simulink model "LinearMPCsiso"  (R2020b)
settings: Solver=FixedStepDiscrete  StartTime=0.0  StopTime=10.0  FixedStep=0.05  RelTol=1e-3
settings Model: Creator=iris  LastModifiedBy=iris
settings DebuggingCC: SFMachineParentedDataDiag=error

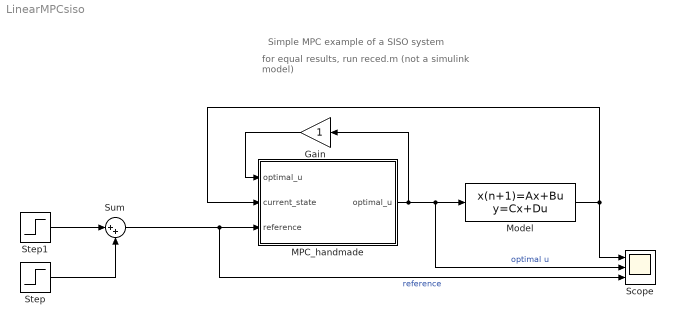
== system LinearMPCsiso ==
  note: for equal results, run reced.m (not a simulink model)
  note: Simple MPC example of a SISO system
  Gain : Gain
  MPC_handmade : MATLAB Function  TreatAsAtomicUnit=on
  Model : DiscreteStateSpace  A=[1 1;0 1]  B=[0.5;1]  C=[1 0;0 1]  D=zeros(2,1)  InitialCondition=[0 0]  SampleTime=-1
  Scope : Scope  NumInputPorts=3
  Step : Step  Time=2  SampleTime=0
  Step1 : Step  Time=5  After=0  SampleTime=0
  Sum : Sum  Inputs=|++
  wires:
  Model/1 -> MPC_handmade/2(current_state), Scope/1
  MPC_handmade/1(optimal_u) -> Gain/1, Scope/2, Model/1  "optimal u"
  Step/1 -> Sum/2
  Step1/1 -> Sum/1
  Sum/1 -> Scope/3, MPC_handmade/3(reference)  "reference"
  Gain/1 -> MPC_handmade/1("optimal_u ")

== matlab function LinearMPCsiso/MPC_handmade ==
  data: optimal_u input; current_state input; reference input; optimal_u output
function optimal_u = MPC_handmade(optimal_u,current_state,reference)
Ap = [1 1 ; 0 1];
Bp = [0.5;1];
Cp = eye(2);
Dp  = zeros(2,1);
Np = 20;
Nc = 4;
% persistent u_next
% if isempty(u_next)
%     u_next = 0;
% end
% MPC gains %%%%%%%%%%%%%%
[m1,n1] = size(Cp);
[n1,n_in] = size(Bp);
A_e = eye(n1+m1,n1+m1);
A_e(1:n1,1:n1) = Ap;
A_e(n1+1:n1+m1,1:n1) = Cp*Ap;
B_e = zeros(n1+m1,n_in);
B_e(1:n1,:) = Bp;
B_e(n1+1:n1+m1,:) = Cp*Bp;
C_e = zeros(m1,n1+m1);
C_e(:,n1+1:n1+m1) = eye(m1,m1);

n = n1+m1;
h = zeros(Np,length(C_e));
F = zeros(Np,size(C_e*A_e,2));
h(1:size(C_e,1),:) = C_e;
F(1:size(C_e,1),:) = C_e*A_e;
for kk = 2:Np
    h(kk,:) = h(kk-1,:)*A_e;
    F(kk,:) = F(kk-1,:)*A_e;
end

v = h*B_e;
Phi = zeros(Np,Nc);
Phi(:,1) = v;
for i=2:Nc 
    Phi(:,i) = [zeros(i-1,1);v(1:Np-i+1,1)]; %Toeplitz matrix
end

BarRs = reference*ones(Np,1);
Phi_Phi = Phi'*Phi;
Phi_F = Phi'*F;
Phi_R = Phi'*BarRs;

%%%%%%%%%%%%%%%%%%%%%%%%%%%%%%%%%%
if isempty(optimal_u)
    u_next = reference;
else
    u_next = optimal_u;
end
 
BarR = 0.5*eye(Nc);
xm_next = Ap*current_state+Bp*u_next;
y_next = xm_next;
Delta_xm = xm_next-current_state;
x_next = [Delta_xm; xm_next];
optimal_DeltaU = inv(Phi_Phi+BarR)*(Phi_R-Phi_F*x_next)
Ky = inv(Phi_Phi+BarR)*(Phi'*F(:,2));
Ky = Ky(1)
Kmpc = inv(Phi_Phi+BarR)*(Phi'*F);
Kmpc = Kmpc(1,:)
eig(A_e-B_e*Kmpc)

u_next = u_next + optimal_DeltaU(1);
optimal_u = u_next;
